simulink model "Copy_of_IpSDKSebesegEsPozicio"  (R2013b)
settings: Solver=FixedStepDiscrete  SolverMode=SingleTasking  StartTime=0.0  StopTime=10.0  FixedStep=1  RelTol=1e-3
undefined symbols (not defined in the file or in its folder): gcbh, xlBlockLoadCallback, xlGetNormalizedPeriod
libraries: xbsIndex_r4 x218
(part 2 of 3)

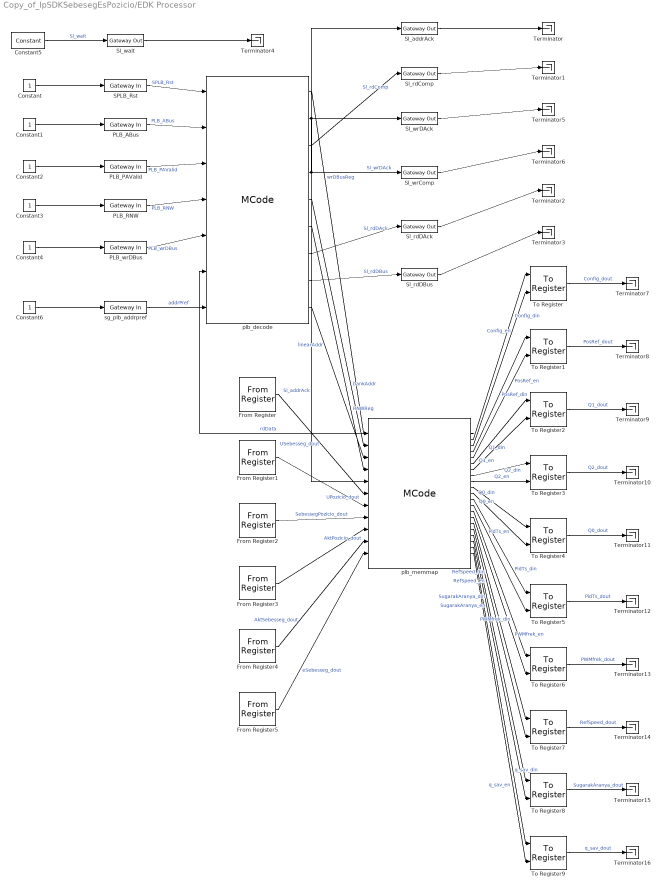
== system Copy_of_IpSDKSebesegEsPozicio/EDK Processor ==
  Constant{,1..4,6} (6 alike) : Constant
  Constant5 : xbsIndex_r4/Constant  const=0  gui_display_data_type=Fixed-point  arith_type=Unsigned  n_bits=1  bin_pt=0  preci_type=Single  exp_width=8  frac_width=24  explicit_period=on  period=xlGetNormalizedPeriod()  equ=P=C  opselect=C  inp2=PCIN>>17  opr=+  inp1=P  carry=CIN  dbl_ovrd=off  block_type=constant
  From Register : xbsIndex_r4/From Register  shared_memory_name='USebesseg'  init=0  period=xlGetNormalizedPeriod()  ownership=Owned and initialized elsewhere  gui_display_data_type=Fixed-point  arith_type="Signed  (2's comp)"  n_bits=32  bin_pt=0  preci_type=Single  dbl_ovrd=off  block_type=fromreg
      settings: AttributesFormatString=<< %<shared_memory_name> >>  infoedit="Register block that reads data to a shared memory register.  Delay of one sample period."
  From Register1 : xbsIndex_r4/From Register  shared_memory_name='UPozicio'  init=0  period=xlGetNormalizedPeriod()  ownership=Owned and initialized elsewhere  gui_display_data_type=Fixed-point  arith_type="Signed  (2's comp)"  n_bits=32  bin_pt=0  preci_type=Single  dbl_ovrd=off  block_type=fromreg
      settings: AttributesFormatString=<< %<shared_memory_name> >>  infoedit="Register block that reads data to a shared memory register.  Delay of one sample period."
  From Register2 : xbsIndex_r4/From Register  shared_memory_name='SebessegPozicio'  init=0  period=xlGetNormalizedPeriod()  ownership=Owned and initialized elsewhere  gui_display_data_type=Fixed-point  arith_type="Signed  (2's comp)"  n_bits=16  bin_pt=0  preci_type=Single  dbl_ovrd=off  block_type=fromreg
      settings: AttributesFormatString=<< %<shared_memory_name> >>  infoedit="Register block that reads data to a shared memory register.  Delay of one sample period."
  From Register3 : xbsIndex_r4/From Register  shared_memory_name='AktPozicio'  init=0  period=xlGetNormalizedPeriod()  ownership=Owned and initialized elsewhere  gui_display_data_type=Fixed-point  arith_type="Signed  (2's comp)"  n_bits=16  bin_pt=0  preci_type=Single  dbl_ovrd=off  block_type=fromreg
      settings: AttributesFormatString=<< %<shared_memory_name> >>  infoedit="Register block that reads data to a shared memory register.  Delay of one sample period."
  From Register4 : xbsIndex_r4/From Register  shared_memory_name='AktSebesseg'  init=0  period=xlGetNormalizedPeriod()  ownership=Owned and initialized elsewhere  gui_display_data_type=Fixed-point  arith_type="Signed  (2's comp)"  n_bits=16  bin_pt=0  preci_type=Single  dbl_ovrd=off  block_type=fromreg
      settings: AttributesFormatString=<< %<shared_memory_name> >>  infoedit="Register block that reads data to a shared memory register.  Delay of one sample period."
  From Register5 : xbsIndex_r4/From Register  shared_memory_name='eSebesseg'  init=0  period=xlGetNormalizedPeriod()  ownership=Owned and initialized elsewhere  gui_display_data_type=Fixed-point  arith_type="Signed  (2's comp)"  n_bits=16  bin_pt=0  preci_type=Single  dbl_ovrd=off  block_type=fromreg
      settings: AttributesFormatString=<< %<shared_memory_name> >>  infoedit="Register block that reads data to a shared memory register.  Delay of one sample period."
  PLB_ABus : xbsIndex_r4/Gateway In  gui_display_data_type=Fixed-point  arith_type=Unsigned  n_bits=32  bin_pt=0  preci_type=Single  exp_width=8  frac_width=24  quantization="Round  (unbiased: +/- Inf)"  overflow=Saturate  period=xlGetNormalizedPeriod()  dbl_ovrd=off  timing_constraint=None  locs_specified=off  LOCs={}  UseAsADC=off  ADCChannel='1'  inherit_from_input=off  hdl_port=on  block_type=gatewayin
      settings: xl_area=[0 0 0 0 32 0 0]  sginterface={'Xilinx'=>{'jtaghwcosim'=>{'non_memory_mapped_port'=>'PLB_ABus'}},'iopad'=>{'constraint'=>'#'}}
  PLB_PAValid : xbsIndex_r4/Gateway In  gui_display_data_type=Fixed-point  arith_type=Unsigned  n_bits=1  bin_pt=0  preci_type=Single  exp_width=8  frac_width=24  quantization="Round  (unbiased: +/- Inf)"  overflow=Saturate  period=xlGetNormalizedPeriod()  dbl_ovrd=off  timing_constraint=None  locs_specified=off  LOCs={}  UseAsADC=off  ADCChannel='1'  inherit_from_input=off  hdl_port=on  block_type=gatewayin
      settings: xl_area=[0 0 0 0 1 0 0]  sginterface={'Xilinx'=>{'jtaghwcosim'=>{'non_memory_mapped_port'=>'PLB_PAValid'}},'iopad'=>{'constraint'=>'#'}}
  PLB_RNW : xbsIndex_r4/Gateway In  gui_display_data_type=Fixed-point  arith_type=Unsigned  n_bits=1  bin_pt=0  preci_type=Single  exp_width=8  frac_width=24  quantization="Round  (unbiased: +/- Inf)"  overflow=Saturate  period=xlGetNormalizedPeriod()  dbl_ovrd=off  timing_constraint=None  locs_specified=off  LOCs={}  UseAsADC=off  ADCChannel='1'  inherit_from_input=off  hdl_port=on  block_type=gatewayin
      settings: xl_area=[0 0 0 0 1 0 0]  sginterface={'Xilinx'=>{'jtaghwcosim'=>{'non_memory_mapped_port'=>'PLB_RNW'}},'iopad'=>{'constraint'=>'#'}}
  PLB_wrDBus : xbsIndex_r4/Gateway In  gui_display_data_type=Fixed-point  arith_type=Unsigned  n_bits=32  bin_pt=0  preci_type=Single  exp_width=8  frac_width=24  quantization="Round  (unbiased: +/- Inf)"  overflow=Saturate  period=xlGetNormalizedPeriod()  dbl_ovrd=off  timing_constraint=None  locs_specified=off  LOCs={}  UseAsADC=off  ADCChannel='1'  inherit_from_input=off  hdl_port=on  block_type=gatewayin
      settings: xl_area=[0 0 0 0 32 0 0]  sginterface={'Xilinx'=>{'jtaghwcosim'=>{'non_memory_mapped_port'=>'PLB_wrDBus'}},'iopad'=>{'constraint'=>'#'}}
  SPLB_Rst : xbsIndex_r4/Gateway In  gui_display_data_type=Fixed-point  arith_type=Unsigned  n_bits=1  bin_pt=0  preci_type=Single  exp_width=8  frac_width=24  quantization="Round  (unbiased: +/- Inf)"  overflow=Saturate  period=xlGetNormalizedPeriod()  dbl_ovrd=off  timing_constraint=None  locs_specified=off  LOCs={}  UseAsADC=off  ADCChannel='1'  inherit_from_input=off  hdl_port=on  block_type=gatewayin
      settings: xl_area=[0 0 0 0 1 0 0]  sginterface={'Xilinx'=>{'jtaghwcosim'=>{'non_memory_mapped_port'=>'SPLB_Rst'}},'iopad'=>{'constraint'=>'#'}}
  Sl_addrAck : xbsIndex_r4/Gateway Out  inherit_from_input=off  hdl_port=on  timing_constraint=None  locs_specified=off  LOCs={}  UseAsDAC=off  DACChannel='1'  block_type=gatewayout
      settings: xl_area=[0 0 0 0 1 0 0]  sginterface={'Xilinx'=>{'jtaghwcosim'=>{'non_memory_mapped_port'=>'Sl_addrAck'}},'iopad'=>{'constraint'=>'#'}}
  Sl_rdComp : xbsIndex_r4/Gateway Out  inherit_from_input=off  hdl_port=on  timing_constraint=None  locs_specified=off  LOCs={}  UseAsDAC=off  DACChannel='1'  block_type=gatewayout
      settings: xl_area=[0 0 0 0 1 0 0]  sginterface={'Xilinx'=>{'jtaghwcosim'=>{'non_memory_mapped_port'=>'Sl_rdComp'}},'iopad'=>{'constraint'=>'#'}}
  Sl_rdDAck : xbsIndex_r4/Gateway Out  inherit_from_input=off  hdl_port=on  timing_constraint=None  locs_specified=off  LOCs={}  UseAsDAC=off  DACChannel='1'  block_type=gatewayout
      settings: xl_area=[0 0 0 0 1 0 0]  sginterface={'Xilinx'=>{'jtaghwcosim'=>{'non_memory_mapped_port'=>'Sl_rdDAck'}},'iopad'=>{'constraint'=>'#'}}
  Sl_rdDBus : xbsIndex_r4/Gateway Out  inherit_from_input=off  hdl_port=on  timing_constraint=None  locs_specified=off  LOCs={}  UseAsDAC=off  DACChannel='1'  block_type=gatewayout
      settings: xl_area=[0 0 0 0 32 0 0]  sginterface={'Xilinx'=>{'jtaghwcosim'=>{'non_memory_mapped_port'=>'Sl_rdDBus'}},'iopad'=>{'constraint'=>'#'}}
  Sl_wait : xbsIndex_r4/Gateway Out  inherit_from_input=off  hdl_port=on  timing_constraint=None  locs_specified=off  LOCs={}  UseAsDAC=off  DACChannel='1'  block_type=gatewayout
      settings: xl_area=[0 0 0 0 1 0 0]  sginterface={'Xilinx'=>{'jtaghwcosim'=>{'non_memory_mapped_port'=>'Sl_wait'}},'iopad'=>{'constraint'=>'#'}}
  Sl_wrComp : xbsIndex_r4/Gateway Out  inherit_from_input=off  hdl_port=on  timing_constraint=None  locs_specified=off  LOCs={}  UseAsDAC=off  DACChannel='1'  block_type=gatewayout
      settings: xl_area=[0 0 0 0 1 0 0]  sginterface={'Xilinx'=>{'jtaghwcosim'=>{'non_memory_mapped_port'=>'Sl_wrComp'}},'iopad'=>{'constraint'=>'#'}}
  Sl_wrDAck : xbsIndex_r4/Gateway Out  inherit_from_input=off  hdl_port=on  timing_constraint=None  locs_specified=off  LOCs={}  UseAsDAC=off  DACChannel='1'  block_type=gatewayout
      settings: xl_area=[0 0 0 0 1 0 0]  sginterface={'Xilinx'=>{'jtaghwcosim'=>{'non_memory_mapped_port'=>'Sl_wrDAck'}},'iopad'=>{'constraint'=>'#'}}
  Terminator{,1..16} (17 alike) : Terminator
  To Register : xbsIndex_r4/To Register  shared_memory_name='Config'  init=0  ownership=Owned and initialized elsewhere  explicit_data_type=on  gui_display_data_type=Fixed-point  arith_type=Unsigned  n_bits=16  bin_pt=0  preci_type=Single  dbl_ovrd=off  block_type=toreg
      settings: AttributesFormatString=<< %<shared_memory_name> >>  infoedit="Register block that writes data to a shared memory register.  Delay of one sample period."
  To Register1 : xbsIndex_r4/To Register  shared_memory_name='PosRef'  init=0  ownership=Owned and initialized elsewhere  explicit_data_type=on  gui_display_data_type=Fixed-point  arith_type="Signed  (2's comp)"  n_bits=16  bin_pt=0  preci_type=Single  dbl_ovrd=off  block_type=toreg
      settings: AttributesFormatString=<< %<shared_memory_name> >>  infoedit="Register block that writes data to a shared memory register.  Delay of one sample period."
  To Register2 : xbsIndex_r4/To Register  shared_memory_name='Q1'  init=0  ownership=Owned and initialized elsewhere  explicit_data_type=on  gui_display_data_type=Fixed-point  arith_type="Signed  (2's comp)"  n_bits=16  bin_pt=0  preci_type=Single  dbl_ovrd=off  block_type=toreg
      settings: AttributesFormatString=<< %<shared_memory_name> >>  infoedit="Register block that writes data to a shared memory register.  Delay of one sample period."
  To Register3 : xbsIndex_r4/To Register  shared_memory_name='Q2'  init=0  ownership=Owned and initialized elsewhere  explicit_data_type=on  gui_display_data_type=Fixed-point  arith_type=Unsigned  n_bits=16  bin_pt=0  preci_type=Single  dbl_ovrd=off  block_type=toreg
      settings: AttributesFormatString=<< %<shared_memory_name> >>  infoedit="Register block that writes data to a shared memory register.  Delay of one sample period."
  To Register4 : xbsIndex_r4/To Register  shared_memory_name='Q0'  init=0  ownership=Owned and initialized elsewhere  explicit_data_type=on  gui_display_data_type=Fixed-point  arith_type="Signed  (2's comp)"  n_bits=16  bin_pt=0  preci_type=Single  dbl_ovrd=off  block_type=toreg
      settings: AttributesFormatString=<< %<shared_memory_name> >>  infoedit="Register block that writes data to a shared memory register.  Delay of one sample period."
  To Register5 : xbsIndex_r4/To Register  shared_memory_name='PidTs'  init=0  ownership=Owned and initialized elsewhere  explicit_data_type=on  gui_display_data_type=Fixed-point  arith_type=Unsigned  n_bits=32  bin_pt=0  preci_type=Single  dbl_ovrd=off  block_type=toreg
      settings: AttributesFormatString=<< %<shared_memory_name> >>  infoedit="Register block that writes data to a shared memory register.  Delay of one sample period."
  To Register6 : xbsIndex_r4/To Register  shared_memory_name='PWMfrek'  init=0  ownership=Owned and initialized elsewhere  explicit_data_type=on  gui_display_data_type=Fixed-point  arith_type=Unsigned  n_bits=16  bin_pt=0  preci_type=Single  dbl_ovrd=off  block_type=toreg
      settings: AttributesFormatString=<< %<shared_memory_name> >>  infoedit="Register block that writes data to a shared memory register.  Delay of one sample period."
  To Register7 : xbsIndex_r4/To Register  shared_memory_name='RefSpeed'  init=0  ownership=Owned and initialized elsewhere  explicit_data_type=on  gui_display_data_type=Fixed-point  arith_type="Signed  (2's comp)"  n_bits=16  bin_pt=0  preci_type=Single  dbl_ovrd=off  block_type=toreg
      settings: AttributesFormatString=<< %<shared_memory_name> >>  infoedit="Register block that writes data to a shared memory register.  Delay of one sample period."
  To Register8 : xbsIndex_r4/To Register  shared_memory_name='SugarakAranya'  init=0  ownership=Owned and initialized elsewhere  explicit_data_type=on  gui_display_data_type=Fixed-point  arith_type="Signed  (2's comp)"  n_bits=16  bin_pt=0  preci_type=Single  dbl_ovrd=off  block_type=toreg
      settings: AttributesFormatString=<< %<shared_memory_name> >>  infoedit="Register block that writes data to a shared memory register.  Delay of one sample period."
  To Register9 : xbsIndex_r4/To Register  shared_memory_name='q_sav'  init=0  ownership=Owned and initialized elsewhere  explicit_data_type=on  gui_display_data_type=Fixed-point  arith_type=Unsigned  n_bits=16  bin_pt=0  preci_type=Single  dbl_ovrd=off  block_type=toreg
      settings: AttributesFormatString=<< %<shared_memory_name> >>  infoedit="Register block that writes data to a shared memory register.  Delay of one sample period."
  plb_decode : xbsIndex_r4/MCode  mfname=xlmax  explicit_period=off  period=1  dbl_ovrd=off  enable_stdout=off  enable_debug=off  mfilecontent=|  suppress_output=on  defparams={}  hide_port_list={}  block_type=mcode
      | function [wrDBusReg, addrAck, rdComp, wrDAck, bankAddr, RNWReg, rdDAck, rdDBus, linearAddr] = plb_bus_decode(plbRst, plbABus, plbPAValid, plbRNW, plbWrDBus, rdData, addrPref)
      | 
      | % constant variables (TODO: should pass from outside)
      | ADDRPREF_LEN = 20;
      | BANKADDR_LEN = 2;
      | LINEARADDR_LEN = 8;
      | ABUS_LEN = 32;
      | DBUS_LEN = 32;
      | 
      | % declare and initialize persistent variables
      | % register input bus signals
      | persistent plbRstReg_, plbRstReg_ = xl_state(0, {xlBoolean});
      | persistent plbABusReg_, plbABusReg_ = xl_state(0, {xlUnsigned, ABUS_LEN, 0});
      | persistent plbPAValidReg_, plbPAValidReg_ = xl_state(0, {xlBoolean});
      | persistent plbRNWReg_, plbRNWReg_ = xl_state(0, {xlUnsigned, 1, 0});
      | persistent plbWrDBusReg_, plbWrDBusReg_ = xl_state(0, {xlUnsigned, DBUS_LEN, 0});
      | 
      | % ===== rest of the outputs =====
      | 
      | bankAddr   = xl_slice(plbABusReg_, 2+BANKADDR_LEN+LINEARADDR_LEN-1, 2+LINEARADDR_LEN);
      | linearAddr = xl_slice(plbABusReg_, 2+LINEARADDR_LEN-1, 2);
      | RNWReg = plbRNWReg_;
      | wrDBusReg = plbWrDBusReg_;
      | 
      | % ===== p_select =====
      | 
      | % register PAValid
      | persistent aValidReg, aValidReg = xl_state(0, {xlBoolean});
      | aValidReg = plbPAValidReg_;
      | 
      | % extract and register the address prefix
      | addrPref_in = xl_slice(plbABusReg_, xl_nbits(plbABusReg_)-1, xl_nbits(plbABusReg_)-ADDRPREF_LEN);
      | if addrPref_in == addrPref
      |     ps1 = true;
      | else 
      |     ps1 = false;
      | end 
      | 
      | persistent ps1Reg, ps1Reg = xl_state(0, ps1);
      | ps1Reg = ps1;
      | 
      | ps = xl_and(ps1Reg, aValidReg);
      | 
      | % ===== addrAck =====
      | 
      | % register ps
      | persistent psReg, psReg = xl_state(0, ps);
      | 
      | addrAck = xfix({xlUnsigned, 1, 0}, xl_and(xl_not(plbRstReg_), ps, xl_not(psReg)));
      | 
      | psReg = ps;
      | 
      | % ===== rdComp, rd/wr DAck =====
      |  
      | rdComp1 = xfix({xlUnsigned, 1, 0}, xl_and(addrAck, RNWReg));
      | 
      | NUM_rdCompDelay = 3;
      | persistent rdCompDelay, rdCompDelay = xl_state(zeros(1, NUM_rdCompDelay), rdComp1, NUM_rdCompDelay);
      | rdComp2 = rdCompDelay.back;
      | rdCompDelay.push_front_pop_back(rdComp1);
      | 
      | persistent rdCompReg, rdCompReg = xl_state(0, rdComp1);
      | rdComp = rdCompReg;
      | rdCompReg = rdComp2;
      | 
      | persistent rdDAckReg, rdDAckReg = xl_state(0, rdComp1);
      | rdDAck = rdDAckReg;
      | rdDAckReg = rdComp;
      | 
      | persistent wrDAckReg, wrDAckReg = xl_state(0, addrAck);
      | wrDAck = wrDAckReg;
      | wrDAckReg = xl_and(addrAck, xl_not(RNWReg));
      | 
      | % ===== rdDBus =====
      | 
      | rdSel = xl_or(rdComp2, rdComp);
      | 
      | if rdSel == 1
      |     rdDBus1 = rdData;
      | else
      |     rdDBus1 = 0;
      | end % if
      | 
      | persistent rdDBusReg, rdDBusReg = xl_state(0, rdDBus1);
      | rdDBus = rdDBusReg;
      | rdDBusReg = rdDBus1;
      | 
      | % rdDBus = xl_concat(rdDBus32, rdDBus32);
      | % rdDBus = rdDBus32;
      | 
      | % ===== update the persistent variables =====
      | 
      | plbRstReg_ = plbRst;
      | plbABusReg_ = plbABus;
      | plbPAValidReg_ = plbPAValid;
      | plbRNWReg_ = plbRNW;
      | plbWrDBusReg_ = xl_slice(plbWrDBus, DBUS_LEN-1, 0);
  plb_memmap : xbsIndex_r4/MCode  mfname=xlmax  explicit_period=off  period=1  dbl_ovrd=off  enable_stdout=off  enable_debug=off  mfilecontent=|  suppress_output=on  defparams={}  hide_port_list={}  block_type=mcode
      | function [read_bank_out, sm_Config_din, sm_Config_en, sm_PosRef_din, sm_PosRef_en, sm_Q1_din, sm_Q1_en, sm_Q2_din, sm_Q2_en, sm_Q0_din, sm_Q0_en, sm_PidTs_din, sm_PidTs_en, sm_PWMfrek_din, sm_PWMfrek_en, sm_RefSpeed_din, sm_RefSpeed_en, sm_SugarakAranya_din, sm_SugarakAranya_en, sm_q_sav_din, sm_q_sav_en] = plb_memmap(wrDBus, bankAddr, linearAddr, RNWReg, addrAck, sm_USebesseg, sm_UPozicio, sm_SebessegPozicio, sm_AktPozicio, sm_AktSebesseg, sm_eSebesseg)
      | 
      | 
      | % connvert the input data to UFix_32_0 (the bus data type)
      | % 'From Register' blocks
      | % sm_USebesseg_bus = xfix({xlUnsigned, 32, 0}, 0);
      | sm_USebesseg_bus = xl_force(sm_USebesseg, xlUnsigned, 0);
      | 
      | % sm_UPozicio_bus = xfix({xlUnsigned, 32, 0}, 0);
      | sm_UPozicio_bus = xl_force(sm_UPozicio, xlUnsigned, 0);
      | 
      | % sm_SebessegPozicio_bus = xfix({xlUnsigned, 32, 0}, 0);
      | sm_SebessegPozicio_bus = xl_force(sm_SebessegPozicio, xlUnsigned, 0);
      | 
      | % sm_AktPozicio_bus = xfix({xlUnsigned, 32, 0}, 0);
      | sm_AktPozicio_bus = xl_force(sm_AktPozicio, xlUnsigned, 0);
      | 
      | % sm_AktSebesseg_bus = xfix({xlUnsigned, 32, 0}, 0);
      | sm_AktSebesseg_bus = xl_force(sm_AktSebesseg, xlUnsigned, 0);
      | 
      | % sm_eSebesseg_bus = xfix({xlUnsigned, 32, 0}, 0);
      | sm_eSebesseg_bus = xl_force(sm_eSebesseg, xlUnsigned, 0);
      | 
      | % 'To Register' blocks
      | 
      | % 'From FIFO' blocks
      | % 'To FIFO' blocks
      | % 'Shared Memory' blocks
      | 
      | % 'dout' ports of 'From Register' blocks
      | 
      | % registered register mux output
      | persistent reg_bank_out_reg; reg_bank_out_reg = xl_state(0, {xlUnsigned, 32, 0});
      | reg_bank_out = reg_bank_out_reg;
      | 
      | if linearAddr == 0
      |     reg_bank_out_reg = sm_USebesseg_bus;
      | elseif linearAddr == 1
      |     reg_bank_out_reg = sm_UPozicio_bus;
      | elseif linearAddr == 2
      |     reg_bank_out_reg = sm_SebessegPozicio_bus;
      | elseif linearAddr == 3
      |     reg_bank_out_reg = sm_AktPozicio_bus;
      | elseif linearAddr == 4
      |     reg_bank_out_reg = sm_AktSebesseg_bus;
      | elseif linearAddr == 5
      |     reg_bank_out_reg = sm_eSebesseg_bus;
      | 
      | end
      | 
      | 
      | % 'From FIFO' and 'To FIFO' blocks
      | 
      | 
      | 
      | 
      | 
      | opCode = xl_concat(addrAck, RNWReg, bankAddr, linearAddr);
      | 
      | % 'Shared Memory' blocks
      | 
      | 
      | 
      | 
      | 
      | % 'din' ports of 'Shared Memory' blocks
      | 
      | 
      | % 'we' ports of 'Shared Memory' blocks
      | 
      | 
      | % 'addr' ports of 'Shared Memory' blocks
      | 
      | 
      | % 're' ports of 'From FIFO' blocks
      | 
      | 
      | % 'en' ports of 'To Register' blocks
      | if opCode == xl_concat(xfix({xlUnsigned, 4, 0}, 10), ...
      |                        xfix({xlUnsigned, xl_nbits(linearAddr), 0}, 0))
      |     sm_Config_en = true;
      | else
      |     sm_Config_en = false;
      | end
      | if opCode == xl_concat(xfix({xlUnsigned, 4, 0}, 10), ...
      |                        xfix({xlUnsigned, xl_nbits(linearAddr), 0}, 1))
      |     sm_PosRef_en = true;
      | else
      |     sm_PosRef_en = false;
      | end
      | if opCode == xl_concat(xfix({xlUnsigned, 4, 0}, 10), ...
      |                        xfix({xlUnsigned, xl_nbits(linearAddr), 0}, 2))
      |     sm_Q1_en = true;
      | else
      |     sm_Q1_en = false;
      | end
      | if opCode == xl_concat(xfix({xlUnsigned, 4, 0}, 10), ...
      |                        xfix({xlUnsigned, xl_nbits(linearAddr), 0}, 3))
      |     sm_Q2_en = true;
      | else
      |     sm_Q2_en = false;
      | end
      | if opCode == xl_concat(xfix({xlUnsigned, 4, 0}, 10), ...
      |                        xfix({xlUnsigned, xl_nbits(linearAddr), 0}, 4))
      |     sm_Q0_en = true;
      | else
      |     sm_Q0_en = false;
      | end
      | if opCode == xl_concat(xfix({xlUnsigned, 4, 0}, 10), ...
      |                        xfix({xlUnsigned, xl_nbits(linearAddr), 0}, 5))
      |     sm_PidTs_en = true;
      | else
      |     sm_PidTs_en = false;
      | end
      | if opCode == xl_concat(xfix({xlUnsigned, 4, 0}, 10), ...
      |                        xfix({xlUnsigned, xl_nbits(linearAddr), 0}, 6))
      |     sm_PWMfrek_en = true;
      | else
      |     sm_PWMfrek_en = false;
      | end
      | if opCode == xl_concat(xfix({xlUnsigned, 4, 0}, 10), ...
      |                        xfix({xlUnsigned, xl_nbits(linearAddr), 0}, 7))
      |     sm_RefSpeed_en = true;
      | else
      |     sm_RefSpeed_en = false;
      | end
      | if opCode == xl_concat(xfix({xlUnsigned, 4, 0}, 10), ...
      |                        xfix({xlUnsigned, xl_nbits(linearAddr), 0}, 8))
      |     sm_SugarakAranya_en = true;
      | else
      |     sm_SugarakAranya_en = false;
      | end
      | if opCode == xl_concat(xfix({xlUnsigned, 4, 0}, 10), ...
      |                        xfix({xlUnsigned, xl_nbits(linearAddr), 0}, 9))
      |     sm_q_sav_en = true;
      | else
      |     sm_q_sav_en = false;
      | end
      | 
      | 
      | % 'din' ports of 'To FIFO' blocks
      | 
      | 
      | % 'we' ports of 'To FIFO' blocks
      | 
      | 
      | % 'din' ports of 'To Register' blocks
      | sm_Config_din = xl_force(xl_slice(wrDBus, 16 - 1, 0), ...
      |                                  xlUnsigned, ...
      |                                  0);
      | sm_PosRef_din = xl_force(xl_slice(wrDBus, 16 - 1, 0), ...
      |                                  xlSigned, ...
      |                                  0);
      | sm_Q1_din = xl_force(xl_slice(wrDBus, 16 - 1, 0), ...
      |                                  xlSigned, ...
      |                                  0);
      | sm_Q2_din = xl_force(xl_slice(wrDBus, 16 - 1, 0), ...
      |                                  xlUnsigned, ...
      |                                  0);
      | sm_Q0_din = xl_force(xl_slice(wrDBus, 16 - 1, 0), ...
      |                                  xlSigned, ...
      |                                  0);
      | sm_PidTs_din = xl_force(xl_slice(wrDBus, 32 - 1, 0), ...
      |                                  xlUnsigned, ...
      |                                  0);
      | sm_PWMfrek_din = xl_force(xl_slice(wrDBus, 16 - 1, 0), ...
      |                                  xlUnsigned, ...
      |                                  0);
      | sm_RefSpeed_din = xl_force(xl_slice(wrDBus, 16 - 1, 0), ...
      |                                  xlSigned, ...
      |                                  0);
      | sm_SugarakAranya_din = xl_force(xl_slice(wrDBus, 16 - 1, 0), ...
      |                                  xlSigned, ...
      |                                  0);
      | sm_q_sav_din = xl_force(xl_slice(wrDBus, 16 - 1, 0), ...
      |                                  xlUnsigned, ...
      |                                  0);
      | 
      | 
      | persistent read_bank_out_reg; read_bank_out_reg = xl_state(0, {xlUnsigned, 32, 0});
      | read_bank_out = read_bank_out_reg;
      | 
      | persistent bankAddr_reg; bankAddr_reg = xl_state(0, bankAddr);
      | 
      | if bankAddr_reg == 0
      |     % Bank 0: Shared Memories
      |     read_bank_out_reg = 0;
      | elseif bankAddr_reg == 1
      |     % Bank 1: From/To FIFOs
      |     read_bank_out_reg =  0;
      | elseif bankAddr_reg == 2
      |     % Bank 2: From/To Registers
      |     read_bank_out_reg = reg_bank_out;
      | elseif bankAddr_reg == 3
      |     % Bank 3: Configuration Registers
      |     read_bank_out_reg = 0;
      | end
      | 
      | bankAddr_reg = bankAddr;
  sg_plb_addrpref : xbsIndex_r4/Gateway In  gui_display_data_type=Fixed-point  arith_type=Unsigned  n_bits=20  bin_pt=0  preci_type=Single  exp_width=8  frac_width=24  quantization="Round  (unbiased: +/- Inf)"  overflow=Saturate  period=xlGetNormalizedPeriod()  dbl_ovrd=off  timing_constraint=None  locs_specified=off  LOCs={}  UseAsADC=off  ADCChannel='1'  inherit_from_input=off  hdl_port=on  block_type=gatewayin
      settings: xl_area=[0 0 0 0 20 0 0]  sginterface={'Xilinx'=>{'jtaghwcosim'=>{'non_memory_mapped_port'=>'sg_plb_addrpref'}},'iopad'=>{'constraint'=>'#'}}
  wires:
  plb_decode/2 -> plb_memmap/5, Sl_addrAck/1  "Sl_addrAck"
  plb_decode/4 -> Sl_wrDAck/1, Sl_wrComp/1  "Sl_wrDAck"
  plb_memmap/21 -> To Register9/2  "q_sav_en"
  plb_memmap/20 -> To Register9/1  "q_sav_din"
  plb_memmap/19 -> To Register8/2  "SugarakAranya_en"
  plb_memmap/18 -> To Register8/1  "SugarakAranya_din"
  plb_memmap/17 -> To Register7/2  "RefSpeed_en"
  plb_memmap/16 -> To Register7/1  "RefSpeed_din"
  plb_memmap/15 -> To Register6/2  "PWMfrek_en"
  plb_memmap/14 -> To Register6/1  "PWMfrek_din"
  plb_memmap/13 -> To Register5/2  "PidTs_en"
  plb_memmap/12 -> To Register5/1  "PidTs_din"
  plb_memmap/11 -> To Register4/2  "Q0_en"
  plb_memmap/10 -> To Register4/1  "Q0_din"
  plb_memmap/9 -> To Register3/2  "Q2_en"
  plb_memmap/8 -> To Register3/1  "Q2_din"
  plb_memmap/7 -> To Register2/2  "Q1_en"
  plb_memmap/6 -> To Register2/1  "Q1_din"
  plb_memmap/5 -> To Register1/2  "PosRef_en"
  plb_memmap/4 -> To Register1/1  "PosRef_din"
  plb_memmap/3 -> To Register/2  "Config_en"
  plb_memmap/2 -> To Register/1  "Config_din"
  plb_memmap/1 -> plb_decode/6  "rdData"
  From Register5/1 -> plb_memmap/11  "eSebesseg_dout"
  From Register4/1 -> plb_memmap/10  "AktSebesseg_dout"
  From Register3/1 -> plb_memmap/9  "AktPozicio_dout"
  From Register2/1 -> plb_memmap/8  "SebessegPozicio_dout"
  From Register1/1 -> plb_memmap/7  "UPozicio_dout"
  From Register/1 -> plb_memmap/6  "USebesseg_dout"
  plb_decode/6 -> plb_memmap/4  "RNWReg"
  plb_decode/9 -> plb_memmap/3  "linearAddr"
  plb_decode/5 -> plb_memmap/2  "bankAddr"
  plb_decode/1 -> plb_memmap/1  "wrDBusReg"
  To Register9/1 -> Terminator16/1  "q_sav_dout"
  To Register8/1 -> Terminator15/1  "SugarakAranya_dout"
  To Register7/1 -> Terminator14/1  "RefSpeed_dout"
  To Register6/1 -> Terminator13/1  "PWMfrek_dout"
  To Register5/1 -> Terminator12/1  "PidTs_dout"
  To Register4/1 -> Terminator11/1  "Q0_dout"
  To Register3/1 -> Terminator10/1  "Q2_dout"
  To Register2/1 -> Terminator9/1  "Q1_dout"
  To Register1/1 -> Terminator8/1  "PosRef_dout"
  To Register/1 -> Terminator7/1  "Config_dout"
  plb_decode/8 -> Sl_rdDBus/1  "Sl_rdDBus"
  plb_decode/7 -> Sl_rdDAck/1  "Sl_rdDAck"
  plb_decode/3 -> Sl_rdComp/1  "Sl_rdComp"
  sg_plb_addrpref/1 -> plb_decode/7  "addrPref"
  PLB_wrDBus/1 -> plb_decode/5  "PLB_wrDBus"
  PLB_RNW/1 -> plb_decode/4  "PLB_RNW"
  PLB_PAValid/1 -> plb_decode/3  "PLB_PAValid"
  PLB_ABus/1 -> plb_decode/2  "PLB_ABus"
  SPLB_Rst/1 -> plb_decode/1  "SPLB_Rst"
  Constant6/1 -> sg_plb_addrpref/1
  Constant5/1 -> Sl_wait/1  "Sl_wait"
  Constant4/1 -> PLB_wrDBus/1
  Constant3/1 -> PLB_RNW/1
  Constant2/1 -> PLB_PAValid/1
  Constant1/1 -> PLB_ABus/1
  Constant/1 -> SPLB_Rst/1
  Sl_wrComp/1 -> Terminator6/1
  Sl_wrDAck/1 -> Terminator5/1
  Sl_wait/1 -> Terminator4/1
  Sl_rdDBus/1 -> Terminator3/1
  Sl_rdDAck/1 -> Terminator2/1
  Sl_rdComp/1 -> Terminator1/1
  Sl_addrAck/1 -> Terminator/1

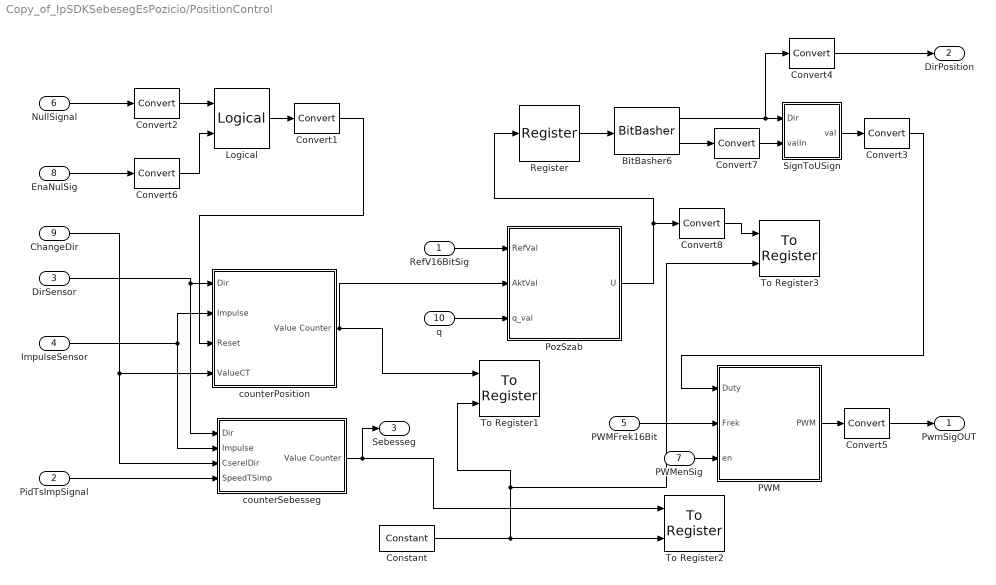
== system Copy_of_IpSDKSebesegEsPozicio/PositionControl ==
  RefV16BitSig : Inport
  PidTsImpSignal : Inport  Port=2
  DirSensor : Inport  Port=3
  ImpulseSensor : Inport  Port=4
  PWMFrek16Bit : Inport  Port=5
  NullSignal : Inport  Port=6
  PWMenSig : Inport  Port=7
  EnaNulSig : Inport  Port=8
  ChangeDir : Inport  Port=9
  q : Inport  Port=10
  BitBasher6 : xbsIndex_r4/BitBasher  bitexpr=|  display_expr=off  sr_1=1  arith_type1=Unsigned  bin_pt1=0  sr_2=2  arith_type2="Signed  (2's comp)"  bin_pt2=0  sr_3=3  arith_type3=Unsigned  bin_pt3=0  sr_4=4  arith_type4=Unsigned  bin_pt4=0  dbl_ovrd=off  block_type=bitbasher
      | <!DOCTYPE HTML PUBLIC "-//W3C//DTD HTML 4.0//EN" "http://www.w3.org/TR/REC-html40/strict.dtd">
      | <html><head><meta name="qrichtext" content="1" /><style type="text/css">
      | p, li { white-space: pre-wrap; }
      | </style></head><body style=" font-family:'MS Shell Dlg 2'; font-size:8.25pt; font-weight:400; font-style:normal;">
      | <p style=" margin-top:12px; margin-bottom:12px; margin-left:0px; margin-right:0px; -qt-block-indent:0; text-indent:0px;"><span style=" font-family:'MS Shell Dlg'; font-size:8pt;">dir={a[16]}<br />val={a[15:0]}</span></p></body></html>
  Constant : xbsIndex_r4/Constant  const=1  gui_display_data_type=Boolean  arith_type=Boolean  n_bits=16  bin_pt=14  preci_type=Single  exp_width=8  frac_width=24  explicit_period=off  period=1  equ=P=C  opselect=C  inp2=PCIN>>17  opr=+  inp1=P  carry=CIN  dbl_ovrd=off  block_type=constant
  Convert1 : xbsIndex_r4/Convert  gui_display_data_type=Fixed-point  arith_type=Unsigned  n_bits=1  bin_pt=0  float_type=Single  exp_bits=8  fraction_bits=24  quantization=Truncate  overflow=Wrap  en=off  latency=0  dbl_ovrd=off  pipeline=off  block_type=convert
  Convert2 : xbsIndex_r4/Convert  gui_display_data_type=Boolean  arith_type=Boolean  n_bits=17  bin_pt=0  float_type=Single  exp_bits=8  fraction_bits=24  quantization=Truncate  overflow=Wrap  en=off  latency=0  dbl_ovrd=off  pipeline=off  block_type=convert
  Convert3 : xbsIndex_r4/Convert  gui_display_data_type=Fixed-point  arith_type=Unsigned  n_bits=16  bin_pt=0  float_type=Single  exp_bits=8  fraction_bits=24  quantization=Truncate  overflow=Wrap  en=off  latency=0  dbl_ovrd=off  pipeline=off  block_type=convert
  Convert4 : xbsIndex_r4/Convert  gui_display_data_type=Boolean  arith_type=Boolean  n_bits=16  bin_pt=0  float_type=Single  exp_bits=8  fraction_bits=24  quantization=Truncate  overflow=Wrap  en=off  latency=0  dbl_ovrd=off  pipeline=off  block_type=convert
  Convert5 : xbsIndex_r4/Convert  gui_display_data_type=Boolean  arith_type=Boolean  n_bits=17  bin_pt=0  float_type=Single  exp_bits=8  fraction_bits=24  quantization=Truncate  overflow=Wrap  en=off  latency=0  dbl_ovrd=off  pipeline=off  block_type=convert
  Convert6 : xbsIndex_r4/Convert  gui_display_data_type=Boolean  arith_type=Boolean  n_bits=17  bin_pt=0  float_type=Single  exp_bits=8  fraction_bits=24  quantization=Truncate  overflow=Wrap  en=off  latency=0  dbl_ovrd=off  pipeline=off  block_type=convert
  Convert7 : xbsIndex_r4/Convert  gui_display_data_type=Fixed-point  arith_type=Unsigned  n_bits=16  bin_pt=0  float_type=Single  exp_bits=8  fraction_bits=24  quantization=Truncate  overflow=Wrap  en=off  latency=0  dbl_ovrd=off  pipeline=off  block_type=convert
  Convert8 : xbsIndex_r4/Convert  gui_display_data_type=Fixed-point  arith_type="Signed  (2's comp)"  n_bits=32  bin_pt=0  float_type=Single  exp_bits=8  fraction_bits=24  quantization=Truncate  overflow=Wrap  en=off  latency=0  dbl_ovrd=off  pipeline=off  block_type=convert
  Logical : xbsIndex_r4/Logical  logical_function=AND  inputs=2  en=off  latency=0  precision=User Defined  arith_type="Signed  (2's comp)"  n_bits=1  bin_pt=0  align_bp=on  dbl_ovrd=off  block_type=logical
  PWM : Subsystem
  PozSzab : Subsystem
  Register : xbsIndex_r4/Register  init=0  rst=off  en=off  dbl_ovrd=off  block_type=register
  SignToUSign : Subsystem
  To Register1 : xbsIndex_r4/To Register  shared_memory_name='AktPozicio'  init=0  ownership=Locally owned and initialized  explicit_data_type=on  gui_display_data_type=Fixed-point  arith_type="Signed  (2's comp)"  n_bits=16  bin_pt=0  preci_type=Single  dbl_ovrd=off  block_type=toreg
      settings: AttributesFormatString=<< %<shared_memory_name> >>  infoedit="Register block that writes data to a shared memory register.  Delay of one sample period."
  To Register2 : xbsIndex_r4/To Register  shared_memory_name='SebessegPozicio'  init=0  ownership=Locally owned and initialized  explicit_data_type=on  gui_display_data_type=Fixed-point  arith_type="Signed  (2's comp)"  n_bits=16  bin_pt=0  preci_type=Single  dbl_ovrd=off  block_type=toreg
      settings: AttributesFormatString=<< %<shared_memory_name> >>  infoedit="Register block that writes data to a shared memory register.  Delay of one sample period."
  To Register3 : xbsIndex_r4/To Register  shared_memory_name='UPozicio'  init=0  ownership=Locally owned and initialized  explicit_data_type=on  gui_display_data_type=Fixed-point  arith_type="Signed  (2's comp)"  n_bits=32  bin_pt=0  preci_type=Single  dbl_ovrd=off  block_type=toreg
      settings: AttributesFormatString=<< %<shared_memory_name> >>  infoedit="Register block that writes data to a shared memory register.  Delay of one sample period."  xl_use_area=on  xl_area=[100,0,0,0,0,0,0]
  counterPosition : Subsystem
  counterSebesseg : Subsystem
  PwmSigOUT : Outport
  DirPosition : Outport  Port=2
  Sebesseg : Outport  Port=3
  wires:
  PWM/1(PWM) -> Convert5/1
  BitBasher6/1 -> SignToUSign/1(Dir), Convert4/1
  BitBasher6/2 -> Convert7/1
  SignToUSign/1(val) -> Convert3/1
  PozSzab/1(U) -> Register/1, Convert8/1
  Convert3/1 -> PWM/1(Duty)
  Convert7/1 -> SignToUSign/2(valIn)
  RefV16BitSig/1 -> PozSzab/1(RefVal)
  DirSensor/1 -> counterSebesseg/1(Dir), counterPosition/1(Dir)
  ImpulseSensor/1 -> counterPosition/2(Impulse), counterSebesseg/2(Impulse)
  PWMFrek16Bit/1 -> PWM/2(Frek)
  PWMenSig/1 -> PWM/3(en)
  Convert5/1 -> PwmSigOUT/1
  Logical/1 -> Convert1/1
  Convert6/1 -> Logical/2
  NullSignal/1 -> Convert2/1
  Convert1/1 -> counterPosition/3(Reset)
  EnaNulSig/1 -> Convert6/1
  Convert2/1 -> Logical/1
  Convert4/1 -> DirPosition/1
  ChangeDir/1 -> counterSebesseg/3(CserelDir), counterPosition/4(ValueCT)
  counterPosition/1(Value Counter) -> PozSzab/2(AktVal), To Register1/1
  q/1 -> PozSzab/3(q_val)
  counterSebesseg/1(Value Counter) -> Sebesseg/1, To Register2/1
  Constant/1 -> To Register2/2, To Register3/2, To Register1/2
  Convert8/1 -> To Register3/1
  PidTsImpSignal/1 -> counterSebesseg/4(SpeedTSimp)
  Register/1 -> BitBasher6/1

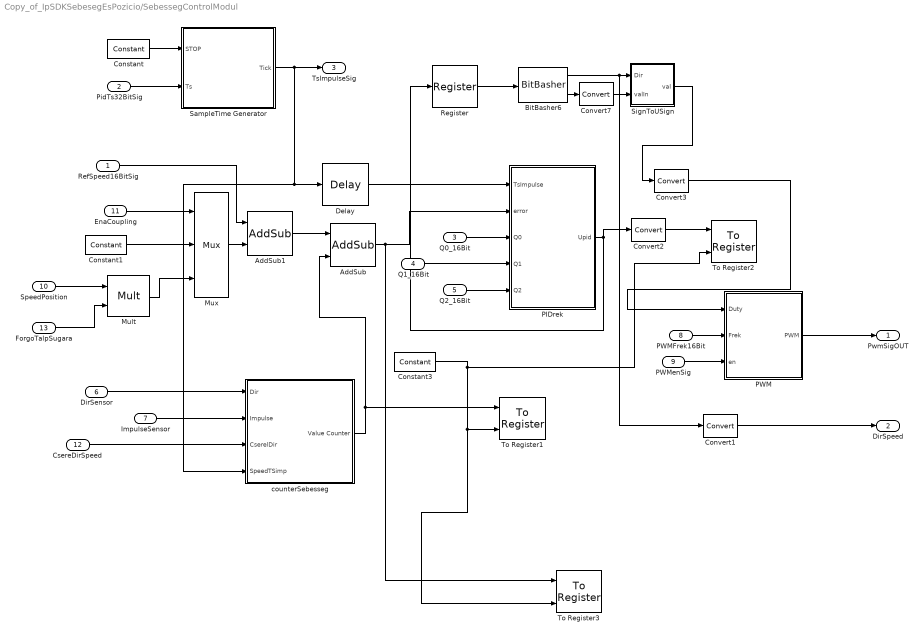
== system Copy_of_IpSDKSebesegEsPozicio/SebessegControlModul ==
  RefSpeed16BitSig : Inport
  PidTs32BitSig : Inport  Port=2
  Q0_16Bit : Inport  Port=3
  Q1_16Bit : Inport  Port=4
  Q2_16Bit : Inport  Port=5
  DirSensor : Inport  Port=6
  ImpulseSensor : Inport  Port=7
  PWMFrek16Bit : Inport  Port=8
  PWMenSig : Inport  Port=9
  SpeedPosition : Inport  Port=10
  EnaCoupling : Inport  Port=11
  CsereDirSpeed : Inport  Port=12
  ForgoTalpSugara : Inport  Port=13
  AddSub : xbsIndex_r4/AddSub  mode=Subtraction  use_carryin=off  use_carryout=off  en=off  latency=0  precision=User Defined  arith_type="Signed  (2's comp)"  n_bits=16  bin_pt=0  quantization=Truncate  overflow=Saturate  dbl_ovrd=off  use_behavioral_HDL=off  hw_selection=Fabric  pipelined=off  block_type=addsub
      settings: xl_use_area=on  xl_area=[10,0,0,0,0,0,0]
  AddSub1 : xbsIndex_r4/AddSub  mode=Subtraction  use_carryin=off  use_carryout=off  en=off  latency=0  precision=User Defined  arith_type="Signed  (2's comp)"  n_bits=16  bin_pt=0  quantization=Truncate  overflow=Saturate  dbl_ovrd=off  use_behavioral_HDL=off  hw_selection=Fabric  pipelined=off  block_type=addsub
  BitBasher6 : xbsIndex_r4/BitBasher  bitexpr=|  display_expr=off  sr_1=1  arith_type1=Unsigned  bin_pt1=0  sr_2=2  arith_type2=Unsigned  bin_pt2=0  sr_3=3  arith_type3=Unsigned  bin_pt3=0  sr_4=4  arith_type4=Unsigned  bin_pt4=0  dbl_ovrd=off  block_type=bitbasher
      | <!DOCTYPE HTML PUBLIC "-//W3C//DTD HTML 4.0//EN" "http://www.w3.org/TR/REC-html40/strict.dtd">
      | <html><head><meta name="qrichtext" content="1" /><style type="text/css">
      | p, li { white-space: pre-wrap; }
      | </style></head><body style=" font-family:'MS Shell Dlg 2'; font-size:8.25pt; font-weight:400; font-style:normal;">
      | <p style=" margin-top:12px; margin-bottom:12px; margin-left:0px; margin-right:0px; -qt-block-indent:0; text-indent:0px;"><span style=" font-family:'MS Shell Dlg'; font-size:8pt;">dir={a[16]}<br />val={a[15:0]}</span></p></body></html>
  Constant : xbsIndex_r4/Constant  const=0  gui_display_data_type=Boolean  arith_type=Boolean  n_bits=16  bin_pt=14  preci_type=Single  exp_width=8  frac_width=24  explicit_period=off  period=1  equ=P=C  opselect=C  inp2=PCIN>>17  opr=+  inp1=P  carry=CIN  dbl_ovrd=off  block_type=constant
  Constant1 : xbsIndex_r4/Constant  const=0  gui_display_data_type=Fixed-point  arith_type=Signed (2's comp)  n_bits=16  bin_pt=0  preci_type=Single  exp_width=8  frac_width=24  explicit_period=off  period=1  equ=P=C  opselect=C  inp2=PCIN>>17  opr=+  inp1=P  carry=CIN  dbl_ovrd=off  block_type=constant
  Constant3 : xbsIndex_r4/Constant  const=1  gui_display_data_type=Boolean  arith_type=Boolean  n_bits=16  bin_pt=14  preci_type=Single  exp_width=8  frac_width=24  explicit_period=off  period=1  equ=P=C  opselect=C  inp2=PCIN>>17  opr=+  inp1=P  carry=CIN  dbl_ovrd=off  block_type=constant
  Convert1 : xbsIndex_r4/Convert  gui_display_data_type=Boolean  arith_type=Boolean  n_bits=16  bin_pt=0  float_type=Single  exp_bits=8  fraction_bits=24  quantization=Truncate  overflow=Wrap  en=off  latency=0  dbl_ovrd=off  pipeline=off  block_type=convert
  Convert2 : xbsIndex_r4/Convert  gui_display_data_type=Fixed-point  arith_type="Signed  (2's comp)"  n_bits=32  bin_pt=0  float_type=Single  exp_bits=8  fraction_bits=24  quantization=Truncate  overflow=Wrap  en=off  latency=0  dbl_ovrd=off  pipeline=off  block_type=convert
  Convert3 : xbsIndex_r4/Convert  gui_display_data_type=Fixed-point  arith_type=Unsigned  n_bits=16  bin_pt=0  float_type=Single  exp_bits=8  fraction_bits=24  quantization=Truncate  overflow=Wrap  en=off  latency=0  dbl_ovrd=off  pipeline=off  block_type=convert
  Convert7 : xbsIndex_r4/Convert  gui_display_data_type=Fixed-point  arith_type=Unsigned  n_bits=16  bin_pt=0  float_type=Single  exp_bits=8  fraction_bits=24  quantization=Truncate  overflow=Wrap  en=off  latency=0  dbl_ovrd=off  pipeline=off  block_type=convert
  Delay : xbsIndex_r4/Delay  rst=off  infoeditControl=Selection of Reset will increase slice count due to use of real FFs and instead of SRLs  en=off  latency=6  dbl_ovrd=off  reg_retiming=off  block_type=delay
      settings: xl_use_area=on  xl_area=[10,0,0,0,0,0,0]
  Mult : xbsIndex_r4/Mult  precision=User Defined  arith_type="Signed  (2's comp)"  n_bits=16  bin_pt=0  quantization=Truncate  overflow=Saturate  en=off  latency=3  dbl_ovrd=off  use_behavioral_HDL=off  opt=Area  use_embedded=on  optimum_pipeline=off  pipeline=on  use_rpm=on  placement_style=Triangular  block_type=mult
  Mux : xbsIndex_r4/Mux  inputs=2  en=off  latency=0  precision=User Defined  arith_type="Signed  (2's comp)"  n_bits=16  bin_pt=0  quantization=Truncate  overflow=Saturate  dbl_ovrd=off  block_type=mux
      settings: xl_use_area=on  xl_area=[1,0,0,0,0,0,0]
  PIDrek : Subsystem
  PWM : Subsystem
  Register : xbsIndex_r4/Register  init=0  rst=off  en=off  dbl_ovrd=off  block_type=register
  SampleTime Generator : Subsystem
  SignToUSign : Subsystem
  To Register1 : xbsIndex_r4/To Register  shared_memory_name='AktSebesseg'  init=0  ownership=Locally owned and initialized  explicit_data_type=on  gui_display_data_type=Fixed-point  arith_type="Signed  (2's comp)"  n_bits=16  bin_pt=0  preci_type=Single  dbl_ovrd=off  block_type=toreg
      settings: AttributesFormatString=<< %<shared_memory_name> >>  infoedit="Register block that writes data to a shared memory register.  Delay of one sample period."
  To Register2 : xbsIndex_r4/To Register  shared_memory_name='USebesseg'  init=0  ownership=Locally owned and initialized  explicit_data_type=on  gui_display_data_type=Fixed-point  arith_type="Signed  (2's comp)"  n_bits=32  bin_pt=0  preci_type=Single  dbl_ovrd=off  block_type=toreg
      settings: AttributesFormatString=<< %<shared_memory_name> >>  infoedit="Register block that writes data to a shared memory register.  Delay of one sample period."
  To Register3 : xbsIndex_r4/To Register  shared_memory_name='eSebesseg'  init=0  ownership=Locally owned and initialized  explicit_data_type=on  gui_display_data_type=Fixed-point  arith_type="Signed  (2's comp)"  n_bits=16  bin_pt=0  preci_type=Single  dbl_ovrd=off  block_type=toreg
      settings: AttributesFormatString=<< %<shared_memory_name> >>  infoedit="Register block that writes data to a shared memory register.  Delay of one sample period."
  counterSebesseg : Subsystem
  PwmSigOUT : Outport
  DirSpeed : Outport  Port=2
  TsImpulseSig : Outport  Port=3
  wires:
  BitBasher6/1 -> SignToUSign/1(Dir), Convert1/1
  BitBasher6/2 -> Convert7/1
  SignToUSign/1(val) -> Convert3/1
  PIDrek/1(Upid) -> Convert2/1, Register/1
  Convert3/1 -> PWM/1(Duty)
  Convert7/1 -> SignToUSign/2(valIn)
  SampleTime Generator/1(Tick) -> TsImpulseSig/1, counterSebesseg/4(SpeedTSimp), Delay/1
  Constant/1 -> SampleTime Generator/1(STOP)
  Delay/1 -> PIDrek/1(TsImpulse)
  PidTs32BitSig/1 -> SampleTime Generator/2(Ts)
  Q2_16Bit/1 -> PIDrek/5(Q2)
  Q1_16Bit/1 -> PIDrek/4(Q1)
  Q0_16Bit/1 -> PIDrek/3(Q0)
  DirSensor/1 -> counterSebesseg/1(Dir)
  ImpulseSensor/1 -> counterSebesseg/2(Impulse)
  PWMFrek16Bit/1 -> PWM/2(Frek)
  PWMenSig/1 -> PWM/3(en)
  PWM/1(PWM) -> PwmSigOUT/1
  Convert1/1 -> DirSpeed/1
  SpeedPosition/1 -> Mult/1
  Mux/1 -> AddSub1/2
  Constant1/1 -> Mux/2
  Mult/1 -> Mux/3
  EnaCoupling/1 -> Mux/1
  ForgoTalpSugara/1 -> Mult/2
  CsereDirSpeed/1 -> counterSebesseg/3(CserelDir)
  counterSebesseg/1(Value Counter) -> To Register1/1, AddSub/2
  Constant3/1 -> To Register2/2, To Register3/2, To Register1/2
  Convert2/1 -> To Register2/1
  AddSub/1 -> To Register3/1, PIDrek/2(error)
  RefSpeed16BitSig/1 -> AddSub1/1
  AddSub1/1 -> AddSub/1
  Register/1 -> BitBasher6/1

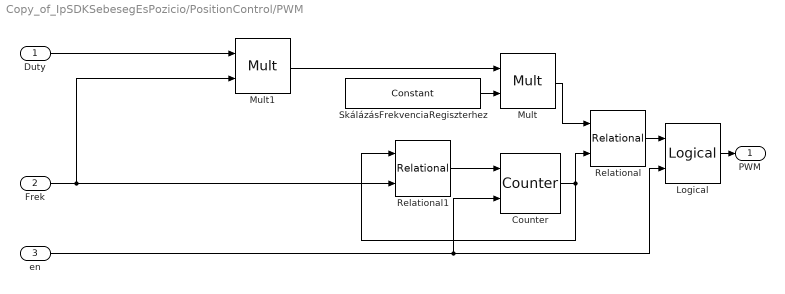
== system Copy_of_IpSDKSebesegEsPozicio/PositionControl/PWM ==
  Duty : Inport
  Frek : Inport  Port=2
  en : Inport  Port=3
  Counter : xbsIndex_r4/Counter  cnt_type=Free Running  cnt_to=Inf  operation=Up  start_count=0  cnt_by_val=1  arith_type=Unsigned  n_bits=16  bin_pt=0  load_pin=off  rst=on  en=on  explicit_period=off  period=2*10^-2  dbl_ovrd=off  use_behavioral_HDL=off  implementation=Fabric  block_type=counter
      settings: xl_use_area=on  xl_area=[1000,0,0,0,0,0,0]
  Logical : xbsIndex_r4/Logical  logical_function=AND  inputs=2  en=off  latency=0  precision=Full  arith_type=Unsigned  n_bits=16  bin_pt=0  align_bp=on  dbl_ovrd=off  block_type=logical
  Mult : xbsIndex_r4/Mult  precision=User Defined  arith_type=Unsigned  n_bits=16  bin_pt=0  quantization=Truncate  overflow=Saturate  en=off  latency=1  dbl_ovrd=off  use_behavioral_HDL=off  opt=Area  use_embedded=on  optimum_pipeline=off  pipeline=on  use_rpm=on  placement_style=Triangular  block_type=mult
      settings: xl_use_area=on  xl_area=[1000,0,0,0,0,0,0]
  Mult1 : xbsIndex_r4/Mult  precision=User Defined  arith_type=Unsigned  n_bits=32  bin_pt=0  quantization=Truncate  overflow=Saturate  en=off  latency=3  dbl_ovrd=off  use_behavioral_HDL=off  opt=Speed  use_embedded=on  optimum_pipeline=off  pipeline=on  use_rpm=on  placement_style=Triangular  block_type=mult
      settings: xl_use_area=on  xl_area=[1000,0,0,0,0,0,0]
  Relational : xbsIndex_r4/Relational  mode=a>b  en=off  latency=0  dbl_ovrd=off  block_type=relational
  Relational1 : xbsIndex_r4/Relational  mode=a=b  en=off  latency=0  dbl_ovrd=off  block_type=relational
  SkálázásFrekvenciaRegiszterhez : xbsIndex_r4/Constant  const=(1/65535) *0.95  gui_display_data_type=Fixed-point  arith_type=Signed (2's comp)  n_bits=32  bin_pt=20  preci_type=Single  exp_width=8  frac_width=24  explicit_period=off  period=1  equ=P=C  opselect=C  inp2=PCIN>>17  opr=+  inp1=P  carry=CIN  dbl_ovrd=off  block_type=constant
  PWM : Outport
  wires:
  Counter/1 -> Relational/2, Relational1/1
  Relational1/1 -> Counter/1
  en/1 -> Logical/2, Counter/2
  Duty/1 -> Mult1/1
  Relational/1 -> Logical/1
  Logical/1 -> PWM/1
  SkálázásFrekvenciaRegiszterhez/1 -> Mult/2
  Mult1/1 -> Mult/1
  Mult/1 -> Relational/1
  Frek/1 -> Mult1/2, Relational1/2
